simulink model "Junctions3_tmp"  (Simulink 8.3)
settings: Solver=ode45  StartTime=0.0  StopTime=10.0  RelTol=1e-3
settings Model: Creator=scaife  LastModifiedBy=bourbouh  CovSFcnEnable=on  ExtModeAutoUpdateStatusClock=off
settings DataIOCC: SignalLoggingName=sigsOut
settings DebuggingCC: SaveWithParameterizedLinksMsg=none  SignalResolutionControl=TryResolveAllWithWarning  SolverPrmCheckMsg=none  MultiTaskDSMMsg=warning  MultiTaskCondExecSysMsg=none  FrameProcessingCompatibilityMsg=error  StateNameClashWarn=none  StrictBusMsg=None
settings HardwareCC: TargetUnknown=on
settings SFSimCC: SimParseCustomCode=off
settings GRTTargetCC: GeneratePreprocessorConditionals=Use local settings

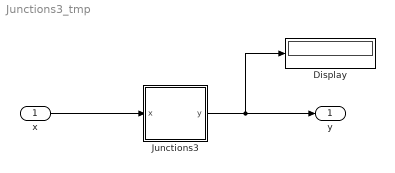
== system Junctions3_tmp ==
  x : Inport
  Display : Display
  Junctions3 : Stateflow chart  TreatAsAtomicUnit=on
      settings: PermitHierarchicalResolution=ParametersOnly
  y : Outport
  wires:
  x/1 -> Junctions3/1(x)
  Junctions3/1(y) -> y/1, Display/1

== stateflow chart Junctions3 ==
  state A
  state B
  (default) -> A
  A -> (junction 7) : [x==0]{y=0}
  (junction 7) -> (junction 8) : [y==0]{y++}
  (junction 8) -> (junction 9) : [y==1]{y++}
  (junction 9) -> (junction 10) : [y==2]{y++}
  (junction 10) -> B : {y++}
  data: x input int32; y output int32 =111111
